simulink model "Follow_Gap_Computation"  (R2023b)
settings: Solver=VariableStepAuto  StartTime=0.0  StopTime=200  RelTol=1e-3
settings Model: Creator=pmodi  LastModifiedBy=pmodi

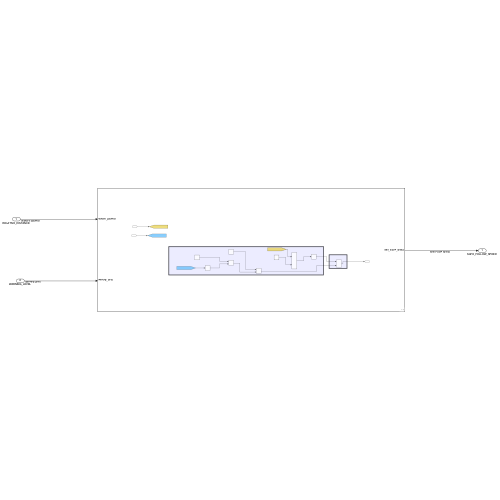
[thumbnail: Simulink's stored preview of the top-level diagram]
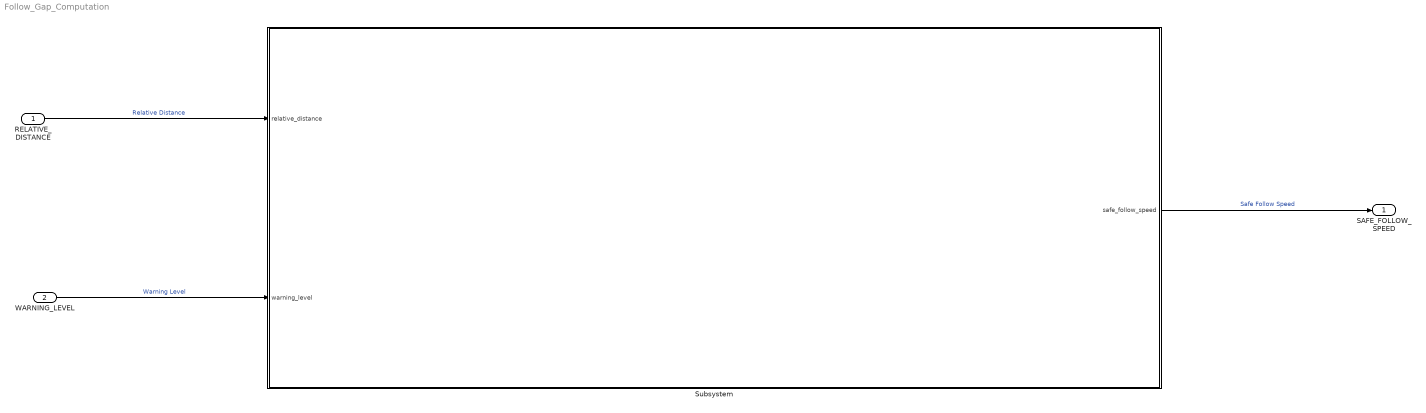
== system Follow_Gap_Computation ==
  RELATIVE_DISTANCE : Inport
  WARNING_LEVEL : Inport  Port=2
  Subsystem : Subsystem
  SAFE_FOLLOW_SPEED : Outport
  wires:
  RELATIVE_DISTANCE/1 -> Subsystem/1(relative_distance)  "Relative Distance"
  WARNING_LEVEL/1 -> Subsystem/2(warning_level)  "Warning Level"
  Subsystem/1(safe_follow_speed) -> SAFE_FOLLOW_SPEED/1  "Safe Follow Speed"

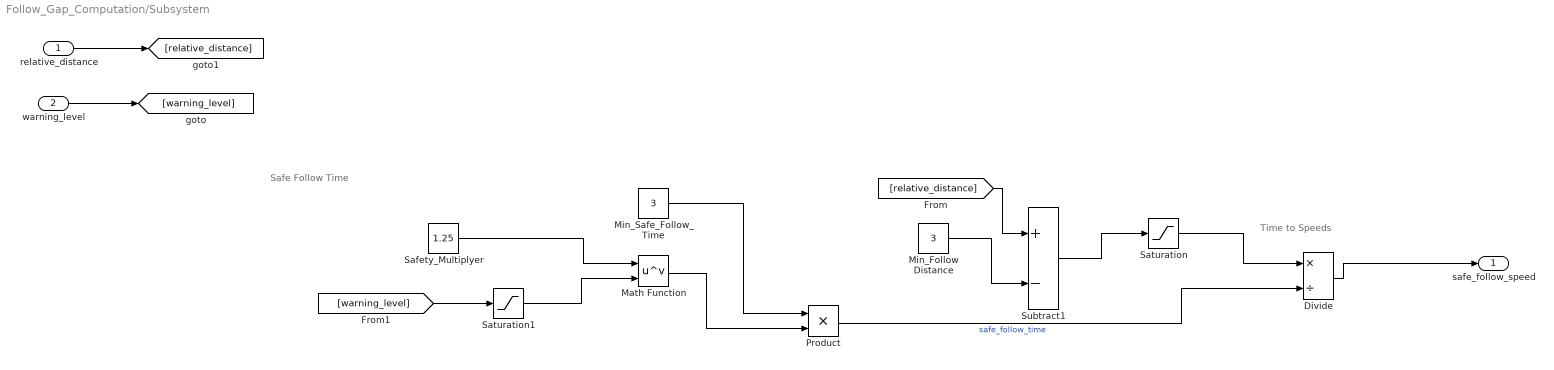
== system Follow_Gap_Computation/Subsystem ==
  note: Time to Speeds
  note: Safe Follow Time
  relative_distance : Inport  Unit=m  LockScale=on
  warning_level : Inport  Port=2  OutMin=0  OutMax=10
  Divide : Product  Inputs=*/
  Math Function : Math  Operator=pow
  Min_Follow Distance : Constant  Value=3
  Min_Safe_Follow_Time : Constant  Value=3
  Product : Product
  Safety_Multiplyer : Constant  Value=1.25
  Saturation : Saturate  UpperLimit=inf  LowerLimit=0
  Saturation1 : Saturate  UpperLimit=10  LowerLimit=0
  Subtract1 : Sum  Inputs=+-
  safe_follow_speed : Outport  OutDataTypeStr=double  Unit=m/s
  wires:
  Subtract1/1 -> Saturation/1
  Divide/1 -> safe_follow_speed/1
  [relative_distance] -> Subtract1/1
  Math Function/1 -> Product/2
  Product/1 -> Divide/2  "safe_follow_time"
  Saturation/1 -> Divide/1
  relative_distance/1 -> [relative_distance]
  Min_Follow Distance/1 -> Subtract1/2
  warning_level/1 -> [warning_level]
  Safety_Multiplyer/1 -> Math Function/1
  Min_Safe_Follow_Time/1 -> Product/1
  [warning_level] -> Saturation1/1
  Saturation1/1 -> Math Function/2
